simulink model "B_6_2012b"  (R2012b)
settings: Solver=ode45  SolverMode=SingleTasking  StartTime=0.0  StopTime=1  MaxStep=1e-4  RelTol=1e-6
StopFcn:
  | %CELEC_plot;
libraries: powerlib x9, simulink x1
settings Model: CovMetricSettings=dwe  CovHtmlReporting=off  covSaveCumulativeToWorkspaceVar=off  CovSaveSingleToWorkspaceVar=off  CovExternalEMLEnable=on  Creator=Administrator  LastModifiedBy=Administrator
settings DataIOCC: LimitDataPoints=off  SaveFormat=StructureWithTime
settings OptimizationCC: ExpressionDepthLimit=128
settings DebuggingCC: UnderspecifiedInitializationDetection=Simplified  MergeDetectMultiDrivingBlocksExec=error  SolverPrmCheckMsg=none  FrameProcessingCompatibilityMsg=error  StateNameClashWarn=none  SFUnexpectedBacktrackingDiag=error  SFNoUnconditionalDefaultTransitionDiag=error
settings HardwareCC: ProdBitPerPointer=64  ProdLargestAtomicFloat=Float  ProdIntDivRoundTo=Zero  ProdEndianess=LittleEndian  ProdHWDeviceType=Specified
settings ModelReferenceCC: PropagateSignalLabelsOutOfModel=on
settings SFSimCC: SimUseLocalCustomCode=on
settings RTWCC: RTWUseLocalCustomCode=on
settings CodeAppCC: CustomSymbolStrType=$N$R$M_T
settings GRTTargetCC: CodeReplacementLibrary=C99 (ISO)  GeneratePreprocessorConditionals=Use local settings

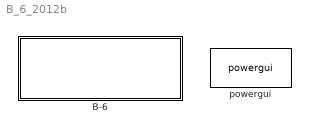
== system B_6_2012b ==
  B-6 : Subsystem  mask{Vset=10, R=2, L=0.02, J=10, KE=1.8, KT=17.2}
      mask prompts: Vset "电源电压(V)"; R "电枢电阻(Ω）"; L "电枢电感(H)"; J "转动惯量(kg.m^3)"; KE "反电势系数(V/rpm)"; KT "电磁转矩系数(N.m/A)"
  powergui : powerlib/powergui  Priority=1  SimulationMode=Continuous  SampleTime=50e-6  frequency=60  Iterations=50  frequencyindice=0  Pbase=100e6  ErrMax=1e-4  UnitsV=kV  UnitsW=MW  buscounter=0  FunctionMessages=off  echomessages=off  EnableUseOfTLC=off  CurrentSourceSwitches=off  DisableSnubberDevices=off  DisableRonSwitches=off  DisableVfSwitches=off  DisplayEquations=off  SolverType=Tustin/Backward Euler (TBE)  Interpol=off  ExternalGateDelay=off  methode=off  Ts=100  x0status=blocks  SPID=on  SwTol=0  HookPort=off  RestoreLinks=warning  ResistiveCurrentMeasurement=off  Frange=[0:2:500]  Ylog=off  Xlog=on  ShowGrid=off  save=off  variable=ZData  structure=0  ZoomFFT=off  StartTime=0.0  cycles=1  DisplayStyle=1  fundamental=60  FreqAxis=off  MaxFrequency=1000  frequencyindicesteady=1  RmsSteady=1  display=off

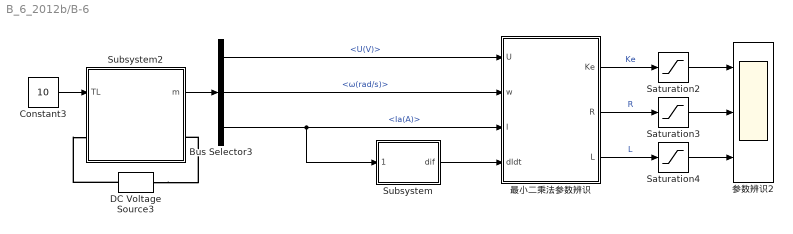
== system B_6_2012b/B-6 ==
  Bus Selector3 : BusSelector  OutputSignals=U(V),ω(rad/s),Ia(A)
  Constant3 : Constant  Value=10
  DC Voltage Source3 : powerlib/Electrical Sources/DC Voltage Source  Amplitude=Vset  Measurements=None
  Saturation2 : Saturate  UpperLimit=5  LowerLimit=0
  Saturation3 : Saturate  UpperLimit=5  LowerLimit=0
  Saturation4 : Saturate  UpperLimit=0.1  LowerLimit=0
  Subsystem : Subsystem
  Subsystem2 : Subsystem
  参数辨识2 : Scope  NumInputPorts=3
      settings: TimeRange=auto  MaxDataPoints=5000  SaveToWorkspace=off  SaveName=ScopeData4  YMin=-0.625~-0.52341~-0.0125  YMax=5.625~4.71068~0.1125  SampleTime=-1
  最小二乘法参数辨识 : MATLAB Function  TreatAsAtomicUnit=on
      settings: PermitHierarchicalResolution=ParametersOnly
  wires:
  Subsystem2/1(m) -> Bus Selector3/1
  Constant3/1 -> Subsystem2/1(TL)
  最小二乘法参数辨识/1(Ke) -> Saturation2/1  "Ke"
  最小二乘法参数辨识/2(R) -> Saturation3/1  "R"
  最小二乘法参数辨识/3(L) -> Saturation4/1  "L"
  Saturation2/1 -> 参数辨识2/1
  Saturation3/1 -> 参数辨识2/2
  Saturation4/1 -> 参数辨识2/3
  Bus Selector3/2 -> 最小二乘法参数辨识/2(w)  "<ω(rad/s)>"
  Bus Selector3/3 -> Subsystem/1(" "), 最小二乘法参数辨识/3(I)  "<Ia(A)>"
  Bus Selector3/1 -> 最小二乘法参数辨识/1(U)  "<U(V)>"
  Subsystem/1(dif) -> 最小二乘法参数辨识/4(dIdt)
  connections:
  DC Voltage Source3/LConn1 -- Subsystem2/RConn1
  DC Voltage Source3/RConn1 -- Subsystem2/LConn1

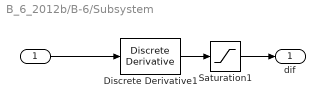
== system B_6_2012b/B-6/Subsystem ==
  " " : Inport
  Discrete Derivative1 : simulink/Discrete/Discrete Derivative  gainval=1.0  ICPrevScaledInput=0  OutMin=[]  OutMax=[]  OutDataType=fixdt(1, 16)  OutScaling=2^-10  DoSatur=off
  Saturation1 : Saturate  UpperLimit=1000  LowerLimit=-1000
  dif : Outport
  wires:
  Discrete Derivative1/1 -> Saturation1/1
  Saturation1/1 -> dif/1
  " "/1 -> Discrete Derivative1/1

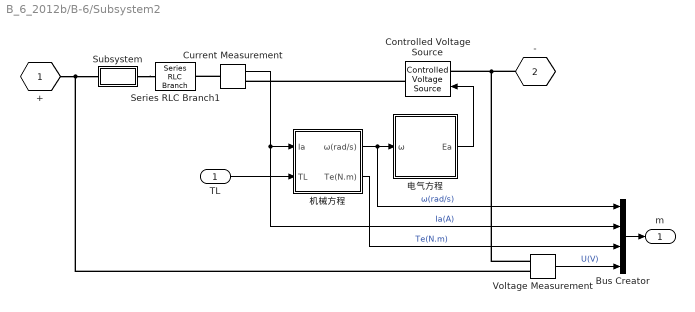
== system B_6_2012b/B-6/Subsystem2 ==
  TL : Inport
  Bus Creator : BusCreator  Inputs=4
  Controlled Voltage Source : powerlib/Electrical Sources/Controlled Voltage Source  Initialize=on  Source_Type=AC  Amplitude=0  Phase=0  Frequency=0  Measurements=None
  Current Measurement : powerlib/Measurements/Current Measurement  PhasorSimulation=off  OutputType=Complex  PSBequivalent=0
  Series RLC Branch1 : powerlib/Elements/Series RLC Branch  LConnTagsString=__new0  RConnTagsString=__new0  BranchType=L  Resistance=R  Inductance=L  SetiL0=off  InitialCurrent=0  Capacitance=1e-6  Setx0=off  InitialVoltage=0  Measurements=None
  Subsystem : Subsystem
  Voltage Measurement : powerlib/Measurements/Voltage Measurement  PhasorSimulation=off  OutputType=Complex  PSBequivalent=0
  机械方程 : Subsystem
  电气方程 : Subsystem
  + : PMIOPort  Tag=PMCPort  Side=Left
  - : PMIOPort  Tag=PMCPort  Port=2  Side=Right
  m : Outport
  wires:
  Current Measurement/1 -> Bus Creator/2, 机械方程/1(Ia)  "Ia(A)"
  TL/1 -> 机械方程/2(TL)
  机械方程/1(ω(rad/s)) -> Bus Creator/1, 电气方程/1(ω)  "ω(rad/s)"
  电气方程/1(Ea) -> Controlled Voltage Source/1
  Bus Creator/1 -> m/1
  机械方程/2(Te(N.m)) -> Bus Creator/3  "Te(N.m)"
  Voltage Measurement/1 -> Bus Creator/4  "U(V)"
  connections:
  Subsystem/RConn1 -- Series RLC Branch1/LConn1
  +/RConn1 -- Voltage Measurement/LConn1 -- Subsystem/LConn1
  Current Measurement/LConn1 -- Series RLC Branch1/RConn1
  Controlled Voltage Source/RConn1 -- Current Measurement/RConn1
  -/RConn1 -- Voltage Measurement/LConn2 -- Controlled Voltage Source/LConn1

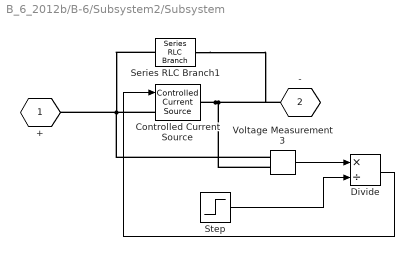
== system B_6_2012b/B-6/Subsystem2/Subsystem ==
  Controlled Current Source : powerlib/Electrical Sources/Controlled Current Source  Initialize=on  Source_Type=AC  Amplitude=0  Phase=0  Frequency=0  Measurements=None
  Divide : Product  Inputs=*/
  Series RLC Branch1 : powerlib/Elements/Series RLC Branch  LConnTagsString=__new0  RConnTagsString=__new0  BranchType=R  Resistance=1e4  Inductance=L  SetiL0=off  InitialCurrent=0  Capacitance=1e-6  Setx0=off  InitialVoltage=0  Measurements=None
  Step : Step  Time=0.5  Before=R  After=R*2  SampleTime=0
  Voltage Measurement3 : powerlib/Measurements/Voltage Measurement  PhasorSimulation=off  OutputType=Complex  PSBequivalent=0
  + : PMIOPort  Tag=PMCPort  Side=Left
  - : PMIOPort  Tag=PMCPort  Port=2  Side=Right
  wires:
  Step/1 -> Divide/2
  Divide/1 -> Controlled Current Source/1
  Voltage Measurement3/1 -> Divide/1
  connections:
  Controlled Current Source/RConn1 -- Series RLC Branch1/RConn1 -- -/RConn1 -- Voltage Measurement3/LConn2
  Controlled Current Source/LConn1 -- Series RLC Branch1/LConn1 -- +/RConn1 -- Voltage Measurement3/LConn1

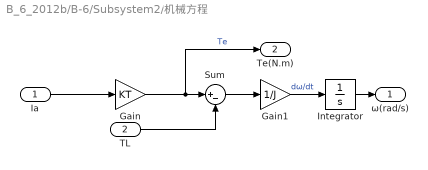
== system B_6_2012b/B-6/Subsystem2/机械方程 ==
  Ia : Inport
  TL : Inport  Port=2
  Gain : Gain  Gain=KT
  Gain1 : Gain  Gain=1/J
  Integrator : Integrator
  Sum : Sum  Inputs=|+-
  ω(rad/s) : Outport
  Te(N.m) : Outport  Port=2
  wires:
  Gain1/1 -> Integrator/1  "dω/dt"
  Sum/1 -> Gain1/1
  Gain/1 -> Te(N.m)/1, Sum/1  "Te"
  TL/1 -> Sum/2
  Ia/1 -> Gain/1
  Integrator/1 -> ω(rad/s)/1

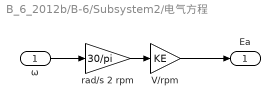
== system B_6_2012b/B-6/Subsystem2/电气方程 ==
  ω : Inport
  V/rpm : Gain  Gain=KE
  rad/s 2 rpm : Gain  Gain=30/pi
  Ea : Outport
  wires:
  rad/s 2 rpm/1 -> V/rpm/1
  ω/1 -> rad/s 2 rpm/1
  V/rpm/1 -> Ea/1

== matlab function B_6_2012b/B-6/最小二乘法参数辨识 ==
  settings: updateMethod=DISCRETE
  data: U input; w input; Ke output; I input; dIdt input; R output; L output
function [Ke,R,L] = CELEC_RLS(U,w,I,dIdt)

persistent P theta P_1 theta_1
if isempty(P_1),          P_1 = 1e4*eye(3); end
if isempty(theta_1),  theta_1 = [0 0 0]'  ; end

r=0.99;
phi = [w*30/pi I dIdt]';
y = U;
K = P_1*phi/(phi'*P_1*phi+r*eye(1));
P = (eye(3)-K*phi')*P_1/r;

e = y - phi'*theta_1;
theta = theta_1 + K*e;

P_1 = P;
theta_1 = theta;

Ke=theta(1);
R =theta(2);
L =theta(3);
end
